simulink model "Lyapunov_order2"  (R2023a)
settings: Solver=FixedStepAuto  StartTime=start_time  StopTime=stop_time  FixedStep=sample_time  RelTol=1e-3
values from neighbouring files (symbols this model uses):
  A = [0 1; 0 1]    [Lyapunov_rule_order2.m]
  Am = [0 1; -2 -3]    [Lyapunov_rule_order2.m]
  B = [0; 1]    [Lyapunov_rule_order2.m]
  D = 0    [Lyapunov_rule_order2.m]
  P = 10*eye(2)    [Lyapunov_rule_order2.m]
settings Model: Creator=Mmoha  LastModifiedBy=Mmoha

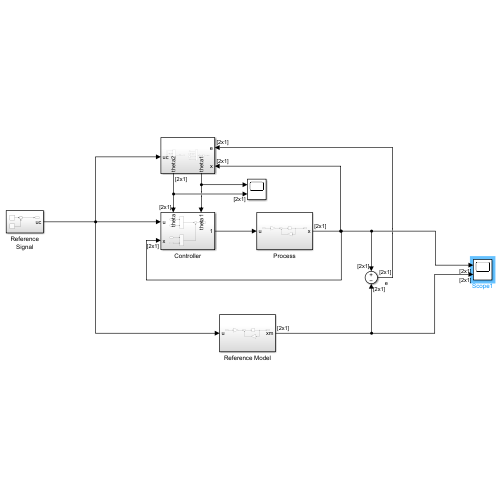
[thumbnail: Simulink's stored preview of the top-level diagram]
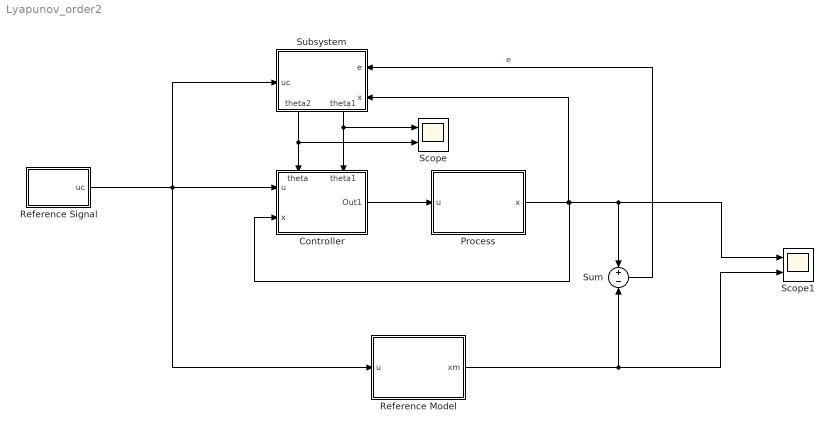
== system Lyapunov_order2 ==
  Controller : Subsystem
      settings: PortSchema="{\"entries\":[{\"content\":{\"sides\":[{\"content\":{\"connectorIds\":[\"In1\",\"In2\"]},\"type\":\"ConnectorPlacement.EquallySpacedRectSide\",\"uuid\":\"19bfb658-27fd-4c0b-8786-eeb0e4dee2ae\"},{\"content\":{\"connectorIds\":[\"Out1\"],\"side\":\"RIGHT\"},\"type\":\"ConnectorPlacement.EquallySpacedRectSide\",\"uuid\":\"360b6564-60bd-491f-8609-763f4a4b58e6\"},{\"content\":{\"connectorIds\":[\"In3\",\"In4\"],\"side\":\"TOP\"},\"type\":\"ConnectorPlacement.EquallySpacedRectSide\",\"uuid\":\"b243d8d4-2ba4-4042-afa8-03d7b661adfb\"}]},\"type\":\"ConnectorPlacement.EquallySpacedConnector\",\"uuid\":\"f7a48170-3b64-4a7a-990b-41657fb93996\"}],\"packageUris\":[\"http://schema.mathworks.com/mf0/Connector/R2020b\"],\"version\":\"1.0\"}"
  Process : Subsystem
  Reference Signal : Subsystem
  Reference Model : Subsystem
  Scope : Scope  NumInputPorts=2
  Scope1 : Scope  NumInputPorts=2
  Subsystem : Subsystem
      settings: PortSchema="{\"entries\":[{\"content\":{\"sides\":[{\"content\":{\"connectorIds\":[\"In1\"]},\"type\":\"ConnectorPlacement.EquallySpacedRectSide\",\"uuid\":\"19bfb658-27fd-4c0b-8786-eeb0e4dee2ae\"},{\"content\":{\"connectorIds\":[\"In2\",\"In3\"],\"side\":\"RIGHT\"},\"type\":\"ConnectorPlacement.EquallySpacedRectSide\",\"uuid\":\"360b6564-60bd-491f-8609-763f4a4b58e6\"},{\"content\":{\"side\":\"TOP\"},\"type\":\"ConnectorPlacement.EquallySpacedRectSide\",\"uuid\":\"b243d8d4-2ba4-4042-afa8-03d7b661adfb\"},{\"content\":{\"connectorIds\":[\"Out1\",\"Out2\"],\"side\":\"BOTTOM\"},\"type\":\"ConnectorPlacement.EquallySpacedRectSide\",\"uuid\":\"2d04a0d8-4dce-4500-be32-805422d5a7ba\"}]},\"type\":\"ConnectorPlacement.EquallySpacedConnector\",\"uuid\":\"f7a48170-3b64-4a7a-990b-41657fb93996\"}],\"packageUris\":[\"http://schema.mathworks.com/mf0/Connector/R2020b\"],\"version\":\"1.0\"}"
  Sum : Sum  Inputs=+|-
  wires:
  Reference Signal/1(uc) -> Subsystem/1(uc), Controller/1(u), Reference Model/1(u)
  Reference Model/1(xm) -> Scope1/2, Sum/2
  Process/1(x) -> Subsystem/3(x), Controller/2(x), Sum/1, Scope1/1
  Controller/1(Out1) -> Process/1(u)
  Sum/1 -> Subsystem/2(e)  "e"
  Subsystem/1(theta2) -> Controller/3(theta), Scope/2
  Subsystem/2(theta1) -> Controller/4(theta1), Scope/1

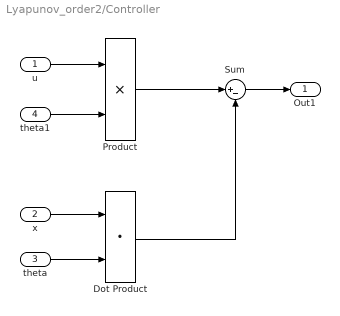
== system Lyapunov_order2/Controller ==
  u : Inport
  x : Inport  Port=2
  theta : Inport  Port=3
  theta1 : Inport  Port=4
  Dot Product : DotProduct  OutDataTypeStr=Inherit: Inherit via internal rule
  Product : Product
  Sum : Sum  Inputs=|+-
  Out1 : Outport
  wires:
  Product/1 -> Sum/1
  u/1 -> Product/1
  x/1 -> Dot Product/1
  theta/1 -> Dot Product/2
  Dot Product/1 -> Sum/2
  Sum/1 -> Out1/1
  theta1/1 -> Product/2

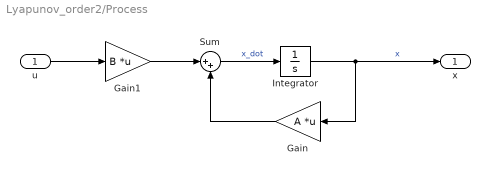
== system Lyapunov_order2/Process ==
  u : Inport
  Gain : Gain  Gain=A  Multiplication=Matrix(K*u)
  Gain1 : Gain  Gain=B  Multiplication=Matrix(K*u)
  Integrator : Integrator  InitialCondition=[0; 0]
  Sum : Sum  Inputs=|++
  x : Outport  PortDimensions=[2 1]
  wires:
  Sum/1 -> Integrator/1  "x_dot"
  Gain1/1 -> Sum/1
  Integrator/1 -> Gain/1, x/1  "x"
  Gain/1 -> Sum/2
  u/1 -> Gain1/1

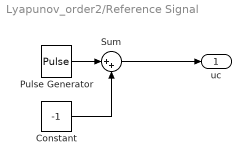
== system Lyapunov_order2/Reference Signal ==
  Constant : Constant  Value=-1
  Pulse Generator : DiscretePulseGenerator  PulseType=Time based  Amplitude=2  Period=20  PulseWidth=50
  Sum : Sum  Inputs=|++
  uc : Outport
  wires:
  Sum/1 -> uc/1
  Pulse Generator/1 -> Sum/1
  Constant/1 -> Sum/2

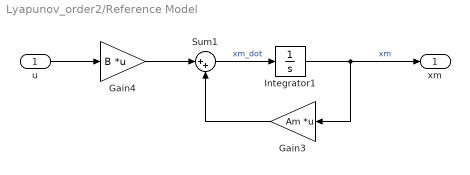
== system Lyapunov_order2/Reference Model ==
  u : Inport
  Gain3 : Gain  Gain=Am  Multiplication=Matrix(K*u)
  Gain4 : Gain  Gain=B  Multiplication=Matrix(K*u)
  Integrator1 : Integrator  InitialCondition=[0; 0]
  Sum1 : Sum  Inputs=|++
  xm : Outport  PortDimensions=[2 1]
  wires:
  Integrator1/1 -> xm/1, Gain3/1  "xm"
  Gain3/1 -> Sum1/2
  Gain4/1 -> Sum1/1
  Sum1/1 -> Integrator1/1  "xm_dot"
  u/1 -> Gain4/1

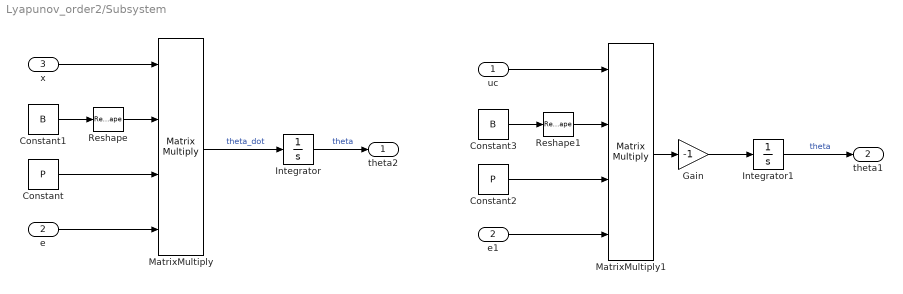
== system Lyapunov_order2/Subsystem ==
  uc : Inport
  e : Inport  Port=2
  x : Inport  Port=3
  Constant : Constant  Value=P
  Constant1 : Constant  Value=B
  Constant2 : Constant  Value=P
  Constant3 : Constant  Value=B
  Gain : Gain  Gain=-1
  Integrator : Integrator
  Integrator1 : Integrator
  MatrixMultiply : Product  Inputs=4  Multiplication=Matrix(*)
  MatrixMultiply1 : Product  Inputs=4  Multiplication=Matrix(*)
  Reshape : Reshape  OutputDimensionality=Row vector (2-D)
  Reshape1 : Reshape  OutputDimensionality=Row vector (2-D)
  e1 : InportShadow  Port=2
  theta2 : Outport
  theta1 : Outport  Port=2
  wires:
  Constant/1 -> MatrixMultiply/3
  MatrixMultiply/1 -> Integrator/1  "theta_dot"
  Constant1/1 -> Reshape/1
  Integrator/1 -> theta2/1  "theta"
  e/1 -> MatrixMultiply/4
  Reshape/1 -> MatrixMultiply/2
  x/1 -> MatrixMultiply/1
  Reshape1/1 -> MatrixMultiply1/2
  Integrator1/1 -> theta1/1  "theta"
  Constant3/1 -> Reshape1/1
  MatrixMultiply1/1 -> Gain/1
  Constant2/1 -> MatrixMultiply1/3
  e1/1 -> MatrixMultiply1/4
  uc/1 -> MatrixMultiply1/1
  Gain/1 -> Integrator1/1
